simulink model "NoiseRemovalAndImageSharpeningHDL"  (R2024b)
settings: Solver=FixedStepDiscrete  StartTime=0.0  StopTime=402*324*10  RelTol=1e-3
undefined symbols (not defined in the file or in its folder): fspecial, gray
libraries: visionhdlio x2, visionhdlfilter x2, visionfilter x1, visionanalysis x1, dspvision x1, visionstatistics x1
settings Model: DataTypeOverride=Off  ModifiedByFormat=The MathWorks, Inc.  SimulationMode=accelerator  Creator=The MathWorks, Inc.  LastModifiedBy=The MathWorks, Inc.
settings SolverCC: AlgebraicLoopSolver=TrustRegion  MinimalZcImpactIntegration=on
settings DataIOCC: LimitDataPoints=on  SaveFormat=Array  SaveOutput=off  SaveTime=off  ReturnWorkspaceOutputs=off
settings OptimizationCC: BlockReduction=off  ConditionallyExecuteInputs=off  DefaultParameterBehavior=Inlined  ReuseModelBlockBuffer=off  LifeSpan=inf
settings DebuggingCC: AlgebraicLoopMsg=error  UnderspecifiedInitializationDetection=Classic  MergeDetectMultiDrivingBlocksExec=none  SolverPrmCheckMsg=warning  SingleTaskRateTransMsg=error  ParameterPrecisionLossMsg=none  UnconnectedInputMsg=warning  UnconnectedOutputMsg=warning  UnconnectedLineMsg=warning  AllowSymbolicDim=off  SFUnexpectedBacktrackingDiag=warning  SFNoUnconditionalDefaultTransitionDiag=warning  SFExecutionAtInitializationDiag=none  ArithmeticOperatorsInVariantConditions=warning
settings HardwareCC: ProdBitPerPointer=32  ProdBitPerSizeT=32  ProdBitPerPtrDiffT=32  ProdLargestAtomicFloat=None  ProdIntDivRoundTo=Undefined  ProdEndianess=Unspecified  ProdWordSize=32  ProdHWDeviceType=ASIC/FPGA->ASIC/FPGA  TargetBitPerLong=64  TargetBitPerPointer=64  TargetBitPerSizeT=64  TargetBitPerPtrDiffT=64  TargetLongLongMode=on  TargetIntDivRoundTo=Zero  TargetEndianess=LittleEndian  TargetWordSize=64  TargetHWDeviceType=Custom Processor->MATLAB Host Computer  ProdEqTarget=off
settings ModelReferenceCC: EnableRefExpFcnMdlSchedulingChecks=on  PropagateSignalLabelsOutOfModel=off
settings SFSimCC: SimUseLocalCustomCode=off  CustomCodeUndefinedFunction=UseInterfaceOnly
settings RTWCC: RTWUseLocalCustomCode=off  GPUComputeCapability=3.5
settings CodeAppCC: StateflowObjectComments=on
settings GRTTargetCC: TargetLangStandard=C89/C90 (ANSI)
settings ConfigComp: CovMetricSettings=dw  CovSaveCumulativeToWorkspaceVar=on  CovSaveSingleToWorkspaceVar=on  CovExternalEMLEnable=off  CovSFcnEnable=off

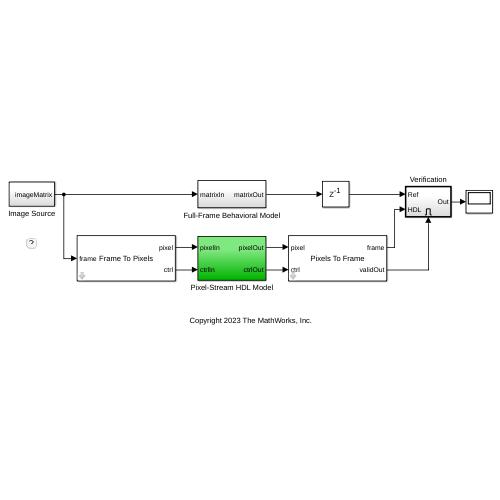
[thumbnail: Simulink's stored preview of the top-level diagram]
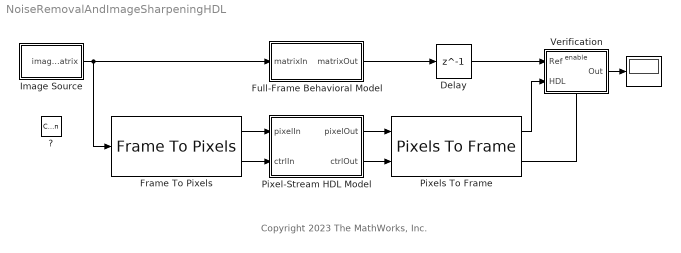
== system NoiseRemovalAndImageSharpeningHDL ==
  note: Copyright 2023 The MathWorks, Inc.
  " " : Display
  "?" : CustomCallbackButton  Configuration="{\"components\":[{\"name\":\"BackgroundImageComponent\",\"settings\":{\"image\":{\"size\":[0,0],\"src\":\"default\",\"srcOrientation\":\"Right\"},\"position\":[0,0,1,1]}},{\"name\":\"ButtonStateComponent\",\"settings\":{\"buttonType\":\"momentary\",\"clickFcn\":\"showExample('visionhdl\\/NoiseRemovalAndImageSharpeningHDLExample')\",\"onValue\":1,\"position\":[0,0,1,1],\"pressDelay\":\"500\",\"pressFcn\":\"\",\"repeatInterval\":\"0\",\"states\":[{\"horizontalAlignment\":\"center\",\"image\":{\"position\":[0,0,1,1],\"src\":\"default\",\"srcOrientation\":\"Right\"},\"label\":{\"color\":[0.01176470588,0.01176470588,0.01176470588,1],\"icon\":{\"size\":[0,0],\"src\":\"default\",\"srcOrientation\":\"Right\"},\"iconPlacement\":\"left\",\"text\":{\"content\":\"?\"}},\"labelOffset\":[0,0],\"verticalAlignment\":\"middle\"},{\"horizontalAlignment\":\"center\",\"image\":{\"position\":[0,0,1,1],\"src\":\"default\",\"srcOrientation\":\"Right\"},\"label\":{\"color\":[0.01176470588,0.01176470588,0.01176470588,1],\"icon\":{\"size\":[0,0],\"src\":\"default\",\"srcOrientation\":\"Right\"},\"iconPlacement\":\"left\",\"text\":{\"content\":\"?\"}},\"labelOffset\":[0,0],\"verticalAlignment\":\"middle\"},{\"horizontalAlignment\":\"center\",\"image\":{\"position\":[0,0,1,1],\"src\":\"default\",\"srcOrientation\":\"Right\"},\"label\":{\"color\":[0.01176470588,0.01176470588,0.01176470588,1],\"icon\":{\"size\":[0,0],\"src\":\"default\",\"srcOrientation\":\"Right\"},\"iconPlacement\":\"left\",\"text\":{\"content\":\"?\"}},\"labelOffset\":[0,0],\"verticalAlignment\":\"middle\"},{\"horizontalAlignment\":\"center\",\"image\":{\"position\":[0,0,1,1],\"src\":\"default\",\"srcOrientation\":\"Right\"},\"label\":{\"color\":[0.01176470588,0.01176470588,0.01176470588,1],\"icon\":{\"size\":[0,0],\"src\":\"default\",\"srcOrientation\":\"Right\"},\"iconPlacement\":\"left\",\"text\":{\"content\":\"?\"}},\"labelOffset\":[0,0],\"verticalAlignment\":\"middle\"}]}},{\"name\":\"ForegroundImageComponent\",\"settings\":{\"image\":{\"size\":[0,0],\"src\":\"default\",\"srcOrientation\":\"Right\"},\"isForeground\":1,\"position\":[0,0,1,1]}}],\"settings\":{\"BindingType\":\"standalone\",\"backgroundColor\":[244,244,244,1],\"backgroundOffset\":0.2,\"backgroundOpacity\":1,\"fixedAspectRatio\":\"off\",\"foregroundColor\":[0.01176470588,0.01176470588,0.01176470588,1],\"migratedFromLegacy\":true,\"useBackgroundColor\":true,\"variant\":\"callback\",\"version\":\"R2023a\"},\"type\":\"Button\"}"  CustomBackgroundColor="{\"color\":[0.9568627451,0.9568627451,0.9568627451],\"show\":true}"
  Delay : Delay  DelayLength=1  InitialCondition=0
  Frame To Pixels : visionhdlio/Frame To Pixels  NumComponents=1  NumPixels=1  VideoFormat=240p  ActivePixelsPerLine=320  ActiveVideoLines=240  TotalPixelsPerLine=402  TotalVideoLines=324  StartingActiveLine=1  FrontPorch=44  SampleTime=0  VideoFormatCache=240p  ActivePixelsPerLineCache=32  ActiveVideoLinesCache=18  TotalPixelsPerLineCache=42  TotalVideoLinesCache=28  StartingActiveLineCache=6  FrontPorchCache=5
  Full-Frame Behavioral Model : Subsystem
  Image Source : Subsystem
  Pixel-Stream HDL Model : Subsystem
  Pixels To Frame : visionhdlio/Pixels To Frame  NumComponents=1  NumPixels=1  VideoFormat=240p  ActivePixelsPerLine=320  ActiveVideoLines=240  TotalPixelsPerLine=402  TotalVideoLines=324  VideoFormatCache=240p  ActivePixelsPerLineCache=32  ActiveVideoLinesCache=18  TotalPixelsPerLineCache=42  TotalVideoLinesCache=28
  Verification : Subsystem
  wires:
  Pixels To Frame/2 -> Verification/Enable
  Image Source/1(imageMatrix) -> Full-Frame Behavioral Model/1(matrixIn), Frame To Pixels/1
  Pixels To Frame/1 -> Verification/2(HDL)
  Verification/1(Out) -> " "/1
  Frame To Pixels/1 -> Pixel-Stream HDL Model/1(pixelIn)
  Frame To Pixels/2 -> Pixel-Stream HDL Model/2(ctrlIn)
  Pixel-Stream HDL Model/2(ctrlOut) -> Pixels To Frame/2
  Pixel-Stream HDL Model/1(pixelOut) -> Pixels To Frame/1
  Full-Frame Behavioral Model/1(matrixOut) -> Delay/1
  Delay/1 -> Verification/1(Ref)

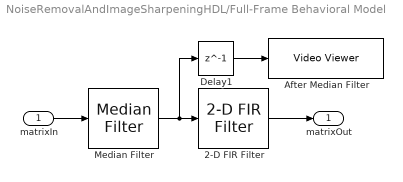
== system NoiseRemovalAndImageSharpeningHDL/Full-Frame Behavioral Model ==
  matrixIn : Inport
  2-D FIR Filter : visionfilter/2-D FIR Filter  separable=off  filtSrc=Specify via dialog  filterMtrx=[0 0 0;0 1 0;0 0 0] - fspecial('laplacian',0.2)  verticalFilter=[4 0]  horizontalFilter=[4 0]  outSize=Same as input port I  padType=Symmetric  padSrc=Specify via dialog  padVal=100  method=Correlation  firstCoeffMode=Binary point scaling  firstCoeffWordLength=17  firstCoeffFracLength=11  firstCoeffSignedness=Signed  firstCoeffLastDataTypeStr=fixdt(1,17,11)  outputSignedness=Auto  accumLastDataTypeStr=Inherit: Same as product output  prodOutputMode=Binary point scaling  prodOutputWordLength=25  prodOutputFracLength=11  prodOutputLastDataTypeStr=fixdt([],25,11)  roundingMode=Round  overflowMode=on  firstCoeffDataTypeStr=fixdt(1,17,11)  firstCoeffMin=[]  firstCoeffMax=[]  prodOutputDataTypeStr=fixdt([],25,11)  accumDataTypeStr=Inherit: Same as product output  outputMin=[]  outputMax=[]
  After Median Filter : VideoViewer  colormapValue=gray(256)  FigPos=[618 589 328 268]
  Delay1 : Delay  DelayLength=1  InitialCondition=0
  Median Filter : visionanalysis/Median Filter  nghbood=[3 3]  outSize=Same as input port I  padType=Replicate  padSrc=Specify via dialog  padVal=0  roundingMode=Floor  overflowMode=off
  matrixOut : Outport  VectorParamsAs1DForOutWhenUnconnected=off
  wires:
  Median Filter/1 -> Delay1/1, 2-D FIR Filter/1
  2-D FIR Filter/1 -> matrixOut/1
  matrixIn/1 -> Median Filter/1
  Delay1/1 -> After Median Filter/1

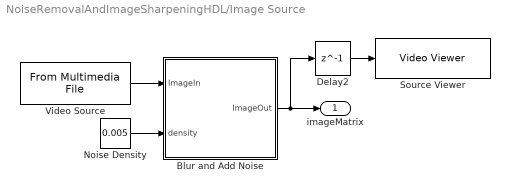
== system NoiseRemovalAndImageSharpeningHDL/Image Source ==
  Blur and Add Noise : MATLAB Function  TreatAsAtomicUnit=on
  Delay2 : Delay  DelayLength=1  InitialCondition=0
  Noise Density : Constant  Value=0.005  OutDataTypeStr=double  SampleTime=402*324
  Source Viewer : VideoViewer  colormapValue=gray(256)  FigPos=[294 589 320 268]
  Video Source : dspvision/From Multimedia File  inputFilename=./fog1v.avi  readRange=[1 Inf]  loop=on  numPlays=inf  outputStreams=Video only  videoDataType=uint8  audioDataType=int16  inheritSampleTime=off  userDefinedSampleTime=324*402  noAudioOutput=off  isIntensityVideo=off  fourcc=Intensity  colorVideoFormat=One multidimensional signal  outputEOF=off  dataOrg=Column-major  audioFrameSize=1024  computeAudioFrameSize=off  outSamplingMode=Sample based
  imageMatrix : Outport  VectorParamsAs1DForOutWhenUnconnected=off
  wires:
  Delay2/1 -> Source Viewer/1
  Noise Density/1 -> Blur and Add Noise/2(density)
  Blur and Add Noise/1(ImageOut) -> imageMatrix/1, Delay2/1
  Video Source/1 -> Blur and Add Noise/1(ImageIn)

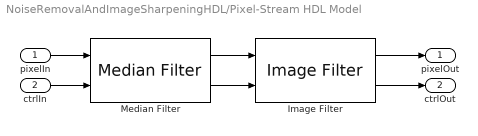
== system NoiseRemovalAndImageSharpeningHDL/Pixel-Stream HDL Model ==
  pixelIn : Inport
  ctrlIn : Inport  Port=2
  Image Filter : visionhdlfilter/Image Filter  CoefficientsSource=Property  Coefficients=[0 0 0;0 1 0;0 0 0] - fspecial('laplacian',0.2)  PaddingMethod=Symmetric  PaddingValue=100  LineBufferSize=2048  SimulateUsing=Code generation  roundingMode=Round  overflowMode=on  CoeffDataTypeStr=fixdt(1,17,11)  CoeffMin=[]  CoeffMax=[]  OutputMin=[]  OutputMax=[]
  Median Filter : visionhdlfilter/Median Filter  NeighborhoodSize=3x3  PaddingMethod=Replicate  PaddingValue=0  LineBufferSize=2048  SimulateUsing=Code generation
  pixelOut : Outport  VectorParamsAs1DForOutWhenUnconnected=off
  ctrlOut : Outport  Port=2  VectorParamsAs1DForOutWhenUnconnected=off
  wires:
  ctrlIn/1 -> Median Filter/2
  pixelIn/1 -> Median Filter/1
  Median Filter/1 -> Image Filter/1
  Image Filter/1 -> pixelOut/1
  Image Filter/2 -> ctrlOut/1
  Median Filter/2 -> Image Filter/2

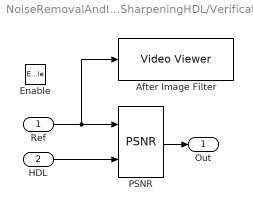
== system NoiseRemovalAndImageSharpeningHDL/Verification ==
  Ref : Inport
  HDL : Inport  Port=2
  Enable : EnablePort
  "After Image Filter " : VideoViewer  colormapValue=gray(256)  FigPos=[950 585 319 264]
  PSNR : visionstatistics/PSNR
  Out : Outport  VectorParamsAs1DForOutWhenUnconnected=off
  wires:
  PSNR/1 -> Out/1
  Ref/1 -> PSNR/1, "After Image Filter "/1
  HDL/1 -> PSNR/2

== matlab function NoiseRemovalAndImageSharpeningHDL/Image Source/Blur and Add Noise ==
  data: ImageIn input; ImageOut output; density input

function ImageOut = fcn(ImageIn, density)	
    ImageOut = cast(zeros(size(ImageIn)),'like', uint8(0)); 
	coder.extrinsic('imnoise'); 
    coeff = fspecial('average',[3 3]);
    ImageBlur = imfilter(ImageIn,coeff);
	ImageOut = imnoise(ImageBlur,'salt & pepper',density);
